simulink model "aerosonde_dynamics_with_autopilot"  (R2021b)
settings: Solver=ode3  StartTime=0.0  StopTime=250  FixedStep=dt  RelTol=1e-6  EnableMultiTasking=on
InitFcn:
  | aerosonde_initialize
  | fault_configurations
  | init_sensor_model
StopFcn:
  | aerosende_grafik;
values from neighbouring files (symbols this model uses):
  aerosonde = AircraftSimData    [aerosonde_data.m]    (also in aerosonde_initialize.m = aerosonde_data)
  aoa_sensor_measurement_limit_rad = deg2rad(30)    [init_sensor_model.m]
  aoa_sensor_noise_power = 0.00030462    [init_sensor_model.m]
  bias_fault_active = TRUE    (= 1)    [fault_configurations.m]
  bias_fault_time = 150    [fault_configurations.m]
  bias_rad = deg2rad(3)    [fault_configurations.m]
  drift_fault_active = FALSE    (= 0)    [fault_configurations.m]
  drift_limit_rad = deg2rad(20)    [fault_configurations.m]
  drift_ratio_rad_s = deg2rad(0.2)    [fault_configurations.m]
  dt = 1/50    (= 0.02)    [aerosonde_initialize.m]
  F = [0 1 0 ... (first row only)    [aerosonde_initialize.m]
  flightconfig = flightconfig_data    [aerosonde_initialize.m]    (also in flightconfig_data.m = siminitialdetails)
  stuck_fault_active = FALSE    (= 0)    [fault_configurations.m]
  x_init = [510.0; -flightconfig.We_VL  ; 0.0]    [aerosonde_initialize.m]
undefined symbols (not defined in the file or in its folder): magnitude, MIL
libraries: simulink_extras x24, simulink x6, aerolibasang x3, aerolibwind2 x3, aerolibbdyn x2, aerolibadyn x1, aerolibtransform2 x1, shareddyn x1, aerolibobsolete x1, sharedutil x1, aerolibatmos2 x1
(part 1 of 2)
settings Model: PacingRate=10  ExtModeTrigDuration=100  Creator=eh3081  LastModifiedBy=altin
settings SolverCC: AlgebraicLoopSolver=TrustRegion
settings DataIOCC: SaveFormat=Array  SignalLoggingSaveFormat=ModelDataLogs  SaveOutput=off  SignalLogging=off  DSMLogging=off  SaveTime=off  StateSaveName=tmp_raccel_xout  SignalLoggingName=tmp_raccel_logsout
settings OptimizationCC: ExpressionDepthLimit=2147483647  InitFltsAndDblsToZero=on  EfficientMapNaN2IntZero=off  LifeSpan=inf
settings DebuggingCC: ReadBeforeWriteMsg=DisableAll  WriteAfterWriteMsg=DisableAll  WriteAfterReadMsg=DisableAll  AlgebraicLoopMsg=none  SaveWithParameterizedLinksMsg=none  UnderspecifiedInitializationDetection=Classic  MergeDetectMultiDrivingBlocksExec=none  SolverPrmCheckMsg=warning  MultiTaskDSMMsg=warning  MultiTaskCondExecSysMsg=none  StateNameClashWarn=warning  SFUnexpectedBacktrackingDiag=warning  SFNoUnconditionalDefaultTransitionDiag=warning  SFExecutionAtInitializationDiag=none  SFMachineParentedDataDiag=warning  ArithmeticOperatorsInVariantConditions=warning
settings HardwareCC: ProdBitPerPointer=32  ProdBitPerSizeT=32  ProdBitPerPtrDiffT=32  ProdLargestAtomicFloat=None  ProdIntDivRoundTo=Undefined  ProdEndianess=Unspecified  ProdWordSize=32  ProdHWDeviceType=32-bit Generic  TargetBitPerPointer=64  TargetBitPerSizeT=64  TargetBitPerPtrDiffT=64  TargetLongLongMode=on  TargetIntDivRoundTo=Zero  TargetEndianess=LittleEndian  TargetWordSize=64  TargetHWDeviceType=MATLAB Host  ProdEqTarget=off
settings ModelReferenceCC: UpdateModelReferenceTargets=IfOutOfDate  PropagateSignalLabelsOutOfModel=off
settings SFSimCC: SFSimEcho=off  SimUseLocalCustomCode=off  CustomCodeUndefinedFunction=UseInterfaceOnly
settings RTWCC: SystemTargetFile=raccel.tlc  TemplateMakefile=raccel_default_tmf  RTWVerbose=off  RTWUseLocalCustomCode=off  RTWUseSimCustomCode=on
settings CodeAppCC: GenerateComments=off  MaxIdLength=128  MangleLength=10  SimulinkBlockComments=off
settings RaccelTargetCC: ParMdlRefBuildCompliant=off  ENABLE_SLEXEC_SSBRIDGE=0  RTWCAPISignals=off  RTWCAPIParams=off  RTWCAPIRootIO=off
settings ConfigComp: CovMetricSettings=dw  CovSaveCumulativeToWorkspaceVar=on  CovSaveSingleToWorkspaceVar=on  CovExternalEMLEnable=off
settings SimscapeCC: SimscapeNormalizeSystem=off
settings ConfigurationSet: Description=SimMechanics 2G

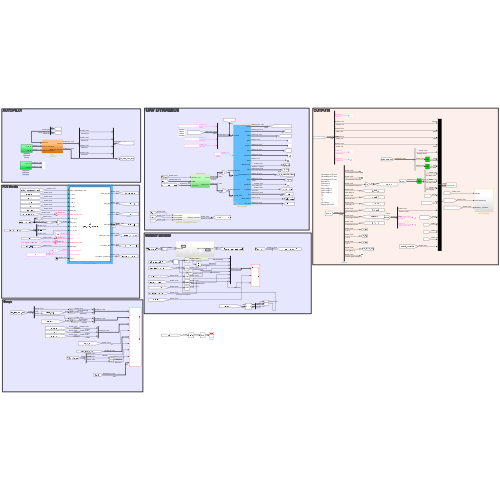
[thumbnail: Simulink's stored preview of the top-level diagram]
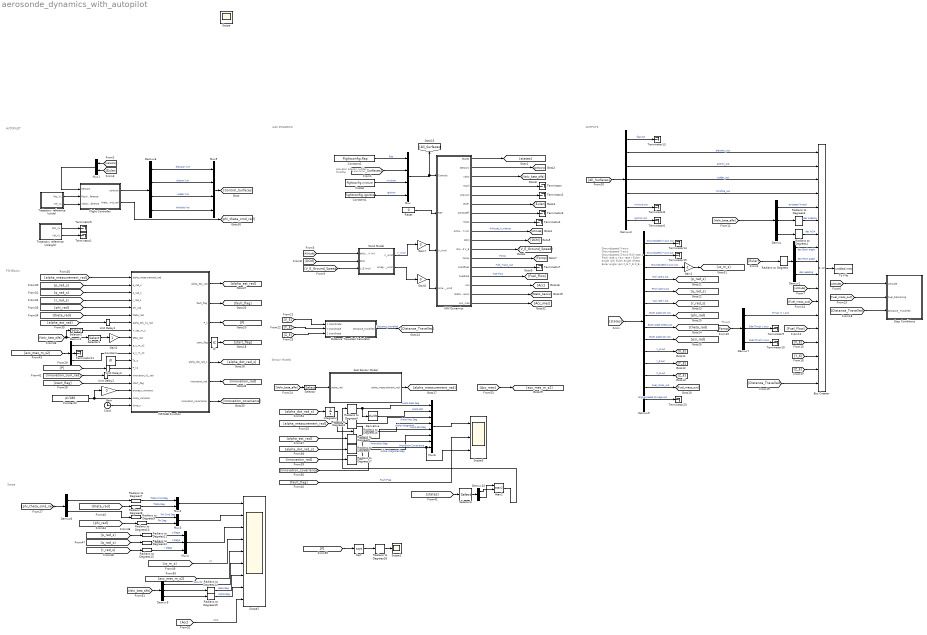
== system aerosonde_dynamics_with_autopilot ==
  note: Scope
  note: FDI Blocks
  note: Sensor Models
  note: AUTOPILOT
  note: OUTPUTS
  note: UAV DYNAMICS
  note: Thrust
  note: elevator
      | aileron
      | rudder
      | throttle
  note: Groundspeed X-axis
      | Groundspeed Y-axis
      | Groundspeed Z-axis
      | Roll rate p
      | Pitch rate q
      | Yaw rate r
      | Euler angle \phi
      | Euler angle \theta
      | Euler angle \psi
      | X_E
      | Y_E
      | Z_E
      | Fuel mass
      | Engine speed \Omega
  " UAV Dynamics" : Subsystem  mask(6-DOF Aerosonde Model){as=aerosonde, Velocities0=flightconfig.velocity_0, Rates0=flightconfig.rates_0, Euler0=flightconfig.euler_0, Position0=flightconfig.position_0, Fuel0=flightconfig.fuel_0, Omega0=flightconfig.Omega_0, GndAlt=0}
      mask prompts: as "Aircraft configuration data:"; Velocities0 "Initial velocity in body axes [u,v,w]: (m/s)"; Rates0 "Initial body rotation rates [p,q,r]: (rad/s)"; Euler0 "Initial Euler orientation [roll, pitch, yaw]: (rad)"; Position0 "Initial position in inertial axes [Xe,Ye,Ze]: (m)"; Fuel0 "Initial fuel mass: (Kg)"; Omega0 "Initial engine speed: (rad/s)"; GndAlt "Ground altitude: (m)"
      mask help:
      | Nonlinear 6-DOF Aerosonde  model with equations of motion in
      | body frame.
      |
      | Version 2011a (18 February 2011)
      mask Help:
      | The block implements the 6-DOF nonlinear Aerosonde model. It is an adaptation of the model provided in the AeroSim blockset. Velocities are computed in body frame.
      | <P><B>Inputs:</B>
      | <LI>Controls = the 4x1 vector of aircraft controls [elevator aileron rudder throttle]. Aerodynamic controls are in radians, throttle is from 0 to 1.</LI>
      | <LI>RST = the integrator reset flag (0 or 1, all integrators on rising edge)
      | <LI>V_wind = the 3x1 vector of background wind speed components in navigation frame [North East Down]</LI>
      | <LI>omega_wind = the 3x1 vector of background wind angular rates in navigation frame [North East Down]</LI>
      | </P>
      | <P><B>Outputs:</B>
      | <LI>States = the 14x1 aircraft state vector [Velocities, Angular rates, Euler angles, Position, Fuel mass, Engine speed].</LI>
      | <LI>Sensors = the 15x1 vector of sensor outputs [GPS Position, GPS Groundspeed, Accelerometers, Gyros, Air data].</LI>
      | <LI>VelW = the 3x1 vector of aircraft velocity in wind axes [Airspeed, sideslip, angle of attack]</LI>
      | <LI>Mach = the Mach number</LI>
      | <LI>Ang Acc = the 3x1 vector of angular accelerations
      | <LI>Euler = the 3x1 vector of Euler angles (roll, pitch, yaw)</LI>
      | <LI>AeroCoeff = the 6x1 vector of aerodynamic coefficients [CD CY CL Cl Cm Cn]</LI>
      | <LI>Mass = the current aircraft mass</LI>
      | <LI>h = the aircraft altitude</LI>
      | </P>
      | <P><B>Parameters:</B>
      | <LI>Aircraft configuration data = structured varaible with aircraft data<BR>
      | obtain by  ``aerosonde=aerosonde_initialize'' for example</LI>
      | <LI>Initial velocities = the 3x1 vector of initial aircraft velocities in body axes [u v w]</LI>
      | <LI>Initial angular rates = the 3x1 vector of initial angular rates [p q r]</LI>
      | <LI>Initial attitude = the 3x1 vector of initial Euler angles [phi theta psi]</LI>
      | <LI>Initial position = the 3x1 vector of initial aircraft location [Lat Lon Alt]</LI>
      | <LI>Initial fuel mass = the initial quantity of fuel on-board the aircraft</LI>
      | <LI>Initial engine speed = the initial engine rotation speed</LI>
      | <LI>Ground altitude = the ground altitude at aircraft location</LI>
      | </P>
      | <P>
      | <I>Version 2010b (26 May 2010)</I>
      | </P>
  AoA Sensor Model : Subsystem
  Atan2 : Trigonometry  Operator=atan2
  Bus Creator : BusCreator  Inputs=18
  Clock : Clock
  Constant : Constant  Value=dt
  Constant1 : Constant  Value=flightconfig.ignition
  Constant2 : Constant  Value=flightconfig.flap
  Constant3 : Constant  Value=pi/180
  Costat : Constant  Value=flightconfig.mixture
  Demux{,1..2,7,9} (5 alike) : Demux  Outputs=3
      Demux settings: DisplayOption=none
      Demux1 settings: DisplayOption=none
  Demux10 : Demux  Outputs=2
  Demux3 : Demux  Outputs=7
  Demux5 : Demux  Outputs=14
  Demux6 : Demux
  Demux8 : Demux  Outputs=2
  Derivative : Derivative
  Distance Travelled Calculator : Subsystem
  Flight Controller : Subsystem
  Gain : Gain  Gain=0
  Gain1 : Gain  Gain=-1
  Gain2 : Gain
  Gain6 : Gain  Gain=0
  Gain7 : Gain  Gain=0
  IC : InitialCondition
  Integrator : Integrator
  MATLAB Function : MATLAB Function  TreatAsAtomicUnit=on
  Mux : Mux  Inputs=[1 4 1 1]
  Mux1 : Mux  Inputs=[15 3]
  Mux2 : Mux  Inputs=2
  Mux3 : Mux  Inputs=2
  Mux4 : Mux  Inputs=3
  Mux5 : Mux
  Mux6 : Mux  Inputs=8
  Radians to Degrees{,1..18} (19 alike) : simulink_extras/Transformations/Radians to Degrees
  Reset : Constant  Value=0
  Scope1 : Scope
  Scope2 : Scope  NumInputPorts=9
  Scope3 : Scope  NumInputPorts=3
  Selector : Selector  InputPortWidth=3  IndexOptions=Index vector (dialog)  Indices=[3]  OutputSizes=1
  Selector1 : Selector  InputPortWidth=3  IndexOptions=Index vector (dialog)  Indices=[2]  OutputSizes=1
  Selector2 : Selector  InputPortWidth=3  IndexOptions=Index vector (dialog)  Indices=[1]  OutputSizes=1
  Selector3 : Selector  InputPortWidth=14  IndexOptions=Index vector (dialog)  Indices=[1 3]  OutputSizes=1
  Sqrt : Sqrt  SaturateOnIntegerOverflow=on
  Stop Conditions : Subsystem
  Terminator{,1..11,13..15,23} (16 alike) : Terminator
  To File : ToFile  MatrixName=fdm  SaveFormat=Timeseries
      settings: Decimation=flightconfig.decimationlogging
  Trajectory reference (circle) : Subsystem
  Trajectory reference (straight) : Subsystem
  Unit Delay1 : UnitDelay  SampleTime=-1  HasFrameUpgradeWarning=on
  Unit Delay2 : UnitDelay  SampleTime=-1  HasFrameUpgradeWarning=on
  Unit Delay3 : UnitDelay  InitialCondition=1e-3  SampleTime=-1  HasFrameUpgradeWarning=on
  Wind Model : Subsystem
  Scope : Scope
  wires:
  Reset/1 -> " UAV Dynamics"/2(RST)
  " UAV Dynamics"/1(States) -> [states]
  Demux/3 -> Radians to Degrees1/1
  Demux/2 -> Radians to Degrees2/1
  Demux/1 -> Bus Creator/5  "airspeed (knots)"
  Radians to Degrees2/1 -> Bus Creator/6  "dec sideslip"
  Radians to Degrees1/1 -> Bus Creator/7  "dec AOA"
  Radians to Degrees/1 -> Demux1/1
  Demux1/2 -> Bus Creator/9  "dec Pitch angle"
  Demux1/3 -> Bus Creator/10  "dec Heading"
  Demux1/1 -> Bus Creator/8  "dec Bank angle"
  Wind Model/1(V_wind) -> Gain7/1  "V_wind"
  Wind Model/2(omega_wind) -> Gain6/1
  " UAV Dynamics"/4(Mach) -> Terminator/1
  " UAV Dynamics"/5(Ang Acc) -> Terminator2/1
  " UAV Dynamics"/7(AeroCoeff) -> Terminator3/1
  " UAV Dynamics"/8(Mass) -> Terminator4/1
  Constant2/1 -> Mux/1  "flap"
  Costat/1 -> Mux/3  "mixture"
  Constant1/1 -> Mux/4  "ignition"
  Mux/1 -> [All_Surfaces], " UAV Dynamics"/1(Controls)
  Flight Controller/1(controls) -> Demux6/1
  Mux1/1 -> Flight Controller/1(Sensors)
  [states] -> Demux5/1
  Trajectory reference (straight)/2(Vel_VL) -> Terminator1/1
  Trajectory reference (straight)/1(Pos_VL) -> Terminator5/1
  Trajectory reference (circle)/2(Vel_VL) -> Flight Controller/3(Velocity reference)
  Demux3/1 -> Terminator13/1  "flap out"
  Demux3/6 -> Terminator8/1  "mixture out"
  Demux3/7 -> Terminator6/1  "ignition out"
  Demux5/1 -> Terminator14/1  "Groundspeed X-axis out"
  Demux5/14 -> Terminator23/1  "Engine speed \\Omega out"
  Demux5/9 -> [psi_rad]  "Euler angle \\psi out"
  Demux5/8 -> [theta_rad]  "Euler angle \\theta out"
  Demux5/7 -> [phi_rad]  "Euler angle \\phi out"
  Demux5/6 -> [r_rad_s]  "Yaw rate r out"
  Demux5/2 -> Terminator15/1  "Groundspeed Y-axis out"
  Demux5/3 -> Gain1/1  "Groundspeed Z-axis out"
  Demux5/4 -> [p_rad_s]  "Roll rate p out"
  Demux5/5 -> [q_rad_s]  "Pitch rate q out"
  Demux5/10 -> [X_E]  "X_E out"
  Demux5/12 -> [Z_E]  "Z_E out"
  Demux6/1 -> Mux5/1  "elevator live"
  Demux6/3 -> Mux5/3  "rudder live"
  Demux6/4 -> Mux5/4  "throttle live"
  Demux7/1 -> Bus Creator/13  "Thrust in x axis"
  Demux7/2 -> Terminator9/1  "Side Thrust y axis"
  Demux7/3 -> Terminator10/1  "Side Thrust z axis"
  Bus Creator/1 -> To File/1
  " UAV Dynamics"/9("Altitude h (m) ") -> [Altitude]  "Altitude_h_metres"
  " UAV Dynamics"/13(OutofFuel) -> Terminator7/1  "Fuel_mass_out"
  Demux3/2 -> Bus Creator/1  "elevator_out"
  Demux3/3 -> Bus Creator/2  "aileron_out"
  Demux3/4 -> Bus Creator/3  "rudder_out"
  Demux3/5 -> Bus Creator/4  "throttle_out"
  Demux5/11 -> [Y_E]  "Y_E out"
  Demux6/2 -> Mux5/2  "aileron live"
  Mux5/1 -> [Control_Surfaces]
  [Control_Surfaces] -> Mux/2
  " UAV Dynamics"/2(Sensors) -> [sensors]
  [sensors] -> Mux1/1
  [Euler] -> Mux1/2
  " UAV Dynamics"/6(Euler) -> [Euler]
  [Euler] -> Radians to Degrees/1
  [Altitude] -> Wind Model/1(altitude h (m))
  [Altitude] -> Bus Creator/11
  [Altitude] -> Stop Conditions/1(Altitude)
  " UAV Dynamics"/10(DCM) -> [DCM]
  [DCM] -> Wind Model/2(DCM)
  " UAV Dynamics"/11(Groundspeed V_E) -> [V_E_Ground_Speed]
  [V_E_Ground_Speed] -> Wind Model/3(V_E (m/s))
  " UAV Dynamics"/12(Fprop) -> [Fprop]  "Fprop"
  [Fprop] -> Demux7/1
  " UAV Dynamics"/3(VelW) -> [Velw_beta_alfa]
  [Velw_beta_alfa] -> Demux/1
  " UAV Dynamics"/14(FuelRate) -> [Fuel_Flow]  "Fuel Flow"
  [Fuel_Flow] -> Bus Creator/14
  Demux5/13 -> [Fuel_mass_out]  "Fuel_mass_out"
  [Fuel_mass_out] -> Stop Conditions/2(Fuel_Remaining)
  [Fuel_mass_out] -> Bus Creator/12
  [X_E] -> Bus Creator/15
  [Y_E] -> Bus Creator/16
  [Z_E] -> Bus Creator/17
  Distance Travelled Calculator/1(Distance_travelled) -> [Distance_Travelled]  "Distance_travelled"
  [Distance_Travelled] -> Stop Conditions/3(Distance_ Travelled)
  [Distance_Travelled] -> Bus Creator/18
  [All_Surfaces] -> Demux3/1
  [X_E] -> Distance Travelled Calculator/1(X Coordinate)
  [Y_E] -> Distance Travelled Calculator/2(Y Coordinate)
  [Z_E] -> Distance Travelled Calculator/3(Z coordinate)
  Trajectory reference (circle)/1(Pos_VL) -> Flight Controller/2(Position reference)
  " UAV Dynamics"/15(" Acc") -> [Acc]
  " UAV Dynamics"/16(Statik_Basinc) -> [Statik_basinc]
  Gain6/1 -> " UAV Dynamics"/4(omega_wind)
  Gain7/1 -> " UAV Dynamics"/3(V_wind)
  [Velw_beta_alfa] -> Selector/1
  Selector/1 -> AoA Sensor Model/1(alpha_rad)
  AoA Sensor Model/1(alpha_measurement_rad) -> [alpha_measurement_rad]
  [alpha_measurement_rad] -> Radians to Degrees3/1
  Radians to Degrees3/1 -> Mux6/3  "Alpha Mes Deg"
  Radians to Degrees4/1 -> Mux6/1, Derivative/1  "Alpha Real Deg"
  [alpha_measurement_rad] -> MATLAB Function/1(alpha_measurement_rad)
  [acc_mes_m_s2] -> Demux2/1
  Demux2/1 -> MATLAB Function/10(a_x_m_s2)
  Demux2/3 -> MATLAB Function/11(a_z_m_s2)
  Constant/1 -> MATLAB Function/12(Ts_s)
  MATLAB Function/4(start_flag) -> IC/1
  IC/1 -> [start_flag]
  [start_flag] -> MATLAB Function/15("start_flag ")
  [P] -> Unit Delay3/1
  Gain/1 -> MATLAB Function/16(process_variance)
  Constant3/1 -> Gain/1, MATLAB Function/17(noise_variance)
  [p_rad_s] -> MATLAB Function/2(p_rad_s)
  [q_rad_s] -> MATLAB Function/3(q_rad_s)
  [r_rad_s] -> MATLAB Function/4(r_rad_s)
  [phi_rad] -> MATLAB Function/5(phi_rad)
  [alpha_est_rad] -> Unit Delay1/1
  MATLAB Function/1(alpha_est_rad) -> [alpha_est_rad]
  MATLAB Function/2(fault_flag) -> [fault_flag]
  [alpha_est_rad] -> Radians to Degrees5/1
  Radians to Degrees5/1 -> Mux6/5  "Alpha Est Deg"
  MATLAB Function/5(alpha_dot_rad_s) -> [alpha_dot_rad_s]
  [alpha_dot_rad_s] -> Radians to Degrees6/1
  Radians to Degrees6/1 -> Mux6/6  "Alpha Integrated Deg"
  Unit Delay1/1 -> MATLAB Function/7(alpha_est_k1_rad)
  [Velw_beta_alfa] -> Selector1/1, Selector2/1
  Selector2/1 -> MATLAB Function/8(V_tas_m_s)
  Demux2/2 -> Terminator11/1
  Selector1/1 -> Gain2/1
  Flight Controller/2(theta_phi_cmd_rad) -> [phi_theta_cmd_rad]
  [phi_theta_cmd_rad] -> Demux8/1
  Demux8/1 -> Radians to Degrees7/1
  Radians to Degrees7/1 -> Mux2/1  "Theta Cmd Deg"
  Radians to Degrees8/1 -> Mux2/2  "Theta Deg"
  Mux2/1 -> Scope2/1
  [theta_rad] -> Radians to Degrees8/1
  Demux8/2 -> Radians to Degrees9/1
  [phi_rad] -> Radians to Degrees10/1
  Radians to Degrees9/1 -> Mux3/1  "Phi Cmd Deg"
  Mux3/1 -> Scope2/2
  [p_rad_s] -> Radians to Degrees11/1
  Radians to Degrees10/1 -> Mux3/2  "Phi Deg"
  [r_rad_s] -> Radians to Degrees13/1
  [q_rad_s] -> Radians to Degrees12/1
  Radians to Degrees11/1 -> Mux4/1  "p Deg/s"
  Radians to Degrees12/1 -> Mux4/2  "q Deg/s"
  Radians to Degrees13/1 -> Mux4/3  "r Deg/s"
  Mux4/1 -> Scope2/3
  Gain1/1 -> [vz_m_s]
  [vz_m_s] -> Scope2/4  "Vz"
  Gain2/1 -> MATLAB Function/9(beta_rad)
  Clock/1 -> MATLAB Function/18(time_s)
  [acc_mes_m_s2] -> Scope2/5
  [Velw_beta_alfa] -> Demux9/1
  Demux9/1 -> Scope2/6  "TAS Kts"
  Demux9/2 -> Radians to Degrees14/1
  Demux9/3 -> Radians to Degrees15/1
  Radians to Degrees14/1 -> Scope2/7  "Beta Deg"
  Radians to Degrees15/1 -> Scope2/8  "Alpha Deg"
  [Acc] -> Scope2/9  "ACC"
  [states] -> Selector3/1
  Selector3/1 -> Demux10/1
  Demux10/2 -> Atan2/1
  Demux10/1 -> Atan2/2
  Atan2/1 -> Radians to Degrees4/1
  " UAV Dynamics"/17(Acc_mes) -> [Acc_mes]
  [Acc_mes] -> [acc_mes_m_s2]
  Derivative/1 -> Mux6/2  "Alpha Dot"
  [alpha_dot_rad_s] -> Integrator/1
  Integrator/1 -> Radians to Degrees16/1
  Radians to Degrees16/1 -> Mux6/4  "Alpha Integrated"
  MATLAB Function/6(innovation_rad) -> [innovation_rad]
  [innovation_rad] -> Radians to Degrees17/1
  Radians to Degrees17/1 -> Mux6/7  "Innovaiton Deg"
  Mux6/1 -> Scope3/1
  [fault_flag] -> Scope3/2  "Fault Flag"
  [innovation_cum_rad] -> Unit Delay2/1
  Unit Delay2/1 -> MATLAB Function/14(innovation_k1_rad)
  MATLAB Function/7(innovation_covariance) -> [innovation_covariance]
  [innovation_covariance] -> Scope3/3, Mux6/8  "Innovaiton Covariance"
  MATLAB Function/3(P_k) -> [P]
  [P] -> Sqrt/1
  [theta_rad] -> MATLAB Function/6(theta_rad)
  Unit Delay3/1 -> MATLAB Function/13(P_k1)
  Radians to Degrees18/1 -> Scope1/1
  Sqrt/1 -> Radians to Degrees18/1

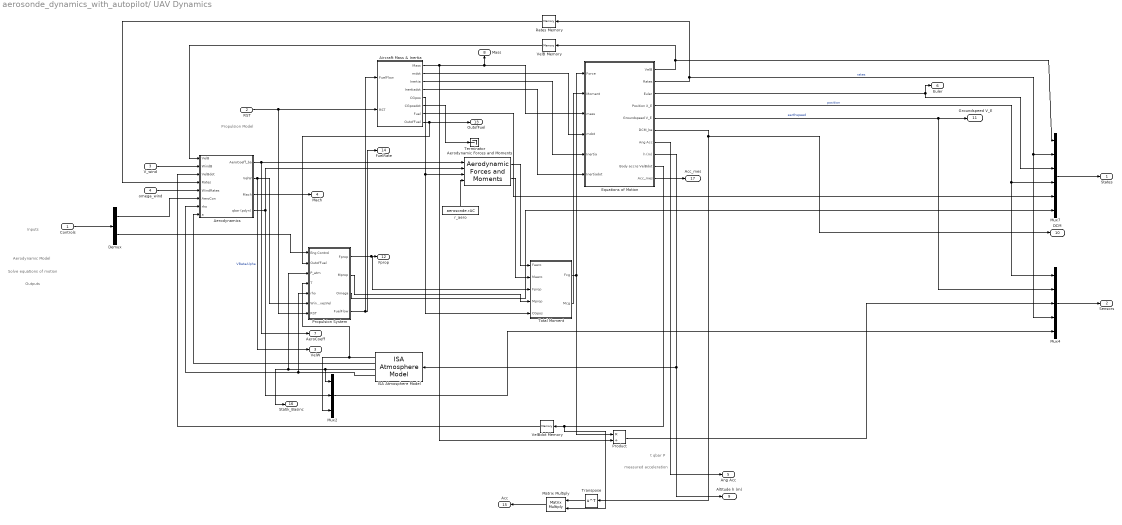
== system aerosonde_dynamics_with_autopilot/ UAV Dynamics ==
  note: t qbar P
  note: measured acceleration
  note: Propulsion Model
  note: Aerodynamic Model
  note: Outputs
  note: Inputs
  note: Solve equations of motion
  Controls : Inport
  RST : Inport  Port=2
  V_wind : Inport  Port=3
  omega_wind : Inport  Port=4
  Aerodynamic Forces and Moments : aerolibadyn/Aerodynamic Forces and Moments   inputAxes=Body  outputForceAxes=Body  outputMomentAxes=Body  S=aerosonde.S  b=aerosonde.b  cbar=aerosonde.c
  Aerodynamics : Subsystem
  Aircraft Mass & Inertia : Subsystem
  Demux : Demux  Outputs=[4,3]
      settings: DisplayOption=none
  Equations of Motion : Subsystem
  ISA Atmosphere Model : aerolibatmos2/ISA Atmosphere Model  custom=off  g=9.80665  gamma=1.4  R=287.0531  L=0.0065  h_trop=11000  h_strat=20000  rho0=1.225  P0=101325  T0=288.15  h0=0
  Matrix Multiply : Product  Multiplication=Matrix(*)
  Mux2 : Mux  Inputs=3
  Mux4 : Mux  Inputs=5
  Mux7 : Mux  Inputs=6
  Product : Product  Inputs=*/  RndMeth=Zero
  Propulsion System : Subsystem  mask(General-aviation propulsion system){OmegaIni=Omega0, RPM=aerosonde.RPM, MAP=aerosonde.MAP, FuelFlow=aerosonde.pFuelFlow, Power=aerosonde.Power, Jeng=aerosonde.Jeng, J=aerosonde.J, CT=aerosonde.CT, CP=aerosonde.CP, Rprop=aerosonde.Rprop, Jprop=aerosonde.Jprop, TSL=aerosonde.TSL}
      mask prompts: OmegaIni "Initial engine speed:"; RPM "Engine RPM vector:"; MAP "Engine MAP vector:"; FuelFlow "Engine fuel flow look-up table:"; Power "Engine power look-up table:"; Jeng "Engine moment of inertia:"; J "Propeller advance ratio vector:"; CT "Propeller coefficient of thrust vector:"; CP "Propeller coefficient of power vector:"; Rprop "Propeller radius:"; Jprop "Propeller moment of inertia:"; TSL "Sea-level temperature:"
      mask help: The block models a general aviation propulsion system including a piston engine and a fixed-pitch propeller.
      mask Help:
      | The block provides a general aviation propulsion system using the AeroSim piston engine and fixed-pitch propeller models.
      | <P><B>Inputs:</B>
      | <LI>Control = the 3x1 engine control vector [Throttle Mixture Ignition]</LI>
      | <LI>OutofFuel = the out-of-fuel flag (0 or 1)</LI>
      | <LI>p = the static pressure at current altitude, in Pa</LI>
      | <LI>T = the air temperature at current altitude, in K</LI>
      | <LI>rho = the air density at current altitude, in kg/m^3</LI>
      | <LI>WindAxesVel = the 3x1 vector of body velocities in wind axes [Airspeed Sideslip Angle-of-attack] in [m/s rad rad]</LI>
      | <LI>RST = the integrator reset flag (rising edge)</LI>
      | </P>
      | <P><B>Output:</B>
      | <LI>Fprop = the 3x1 vector of propulsion system forces applied to the airframe, at the propeller hub location</LI>
      | <LI>Mprop = the 3x1 vector of propulsion system moments applied to the airframe</LI>
      | <LI>Omega = the engine shaft rotation speed, in rad/s</LI>
      | <LI>FuelFlow = the mass fuel flow, in kg/s</LI>
      | <LI>EngCoeff = the 5x1 engine coefficient vector [MAP Airflow Fuelflow BSFC Power] in [kPa kg/s kg/s g/(W*hr) W]</LI>
      | <LI>PropCoeff = the 3x1 propeller coefficient vector [J CT CP]</LI>
      | </P>
      | <P><B>Parameters:</B>
      | <LI>Initial engine speed = the initial value for the engine speed, in rad/s</LI>
      | <LI>RPM vector = the engine speed interpolation vector, in rpm</LI>
      | <LI>MAP vector = the manifold air pressure interpolation vector, in kPa</LI>
      | <LI>Fuel flow = the 2-D look-up table for fuel flow, as function of MAP and RPM, in g/hr</LI>
      | <LI>Power = the 2-D look-up table for power, as function of MAP and RPM, in W</LI>
      | <LI>Engine moment of inertia = the moment of inertia of the rotating engine parts (shaft)</LI>
      | <LI>Advance ratio = the advance ratio vector for interpolation</LI>
      | <LI>Coefficient of thrust = the coefficient of thrust vector for interpolation</LI>
      | <LI>Coefficient of power = the coefficient of power vector for interpolation</LI>
      | <LI>Radius = the propeller radius</LI>
      | <LI>Propeller moment of inertia = the moment of inertia of the propeller</LI>
      | <LI>Sea-level temperature = the ambient temperature for which the above engine look-up tables are given</LI>
      | </P>
  Rates Memory : Memory  InitialCondition=flightconfig.rates_0  LinearizeMemory=on
  Terminator : Terminator
  Total Moment : Subsystem
  Transpose : Math  Operator=transpose  SaturateOnIntegerOverflow=on
  VelB Memory : Memory  InitialCondition=flightconfig.velocity_0  LinearizeMemory=on
  VelBdot Memory : Memory  LinearizeMemory=on
  r_aero : Constant  Value=aerosonde.rAC
  States : Outport
  Sensors : Outport  Port=2
  VelW : Outport  Port=3
  Mach : Outport  Port=4
  Ang Acc : Outport  Port=5
  Euler : Outport  Port=6
  AeroCoeff : Outport  Port=7
  Mass : Outport  Port=8
  "Altitude h (m) " : Outport  Port=9
  DCM : Outport  Port=10
  Groundspeed V_E : Outport  Port=11
  Fprop : Outport  Port=12
  OutofFuel : Outport  Port=13  OutDataTypeStr=boolean
  FuelRate : Outport  Port=14
  " Acc" : Outport  Port=15
  Statik_Basinc : Outport  Port=16
  Acc_mes : Outport  Port=17
  wires:
  Aircraft Mass & Inertia/7(Fuel) -> Mux7/5
  Propulsion System/3(Omega) -> Mux7/6
  ISA Atmosphere Model/4 -> Propulsion System/5(rho), Aerodynamics/7(rho)
  VelB Memory/1 -> Aerodynamics/1(VelB)
  Equations of Motion/6(DCM_be) -> Transpose/1, DCM/1
  Rates Memory/1 -> Aerodynamics/4(Rates)
  Equations of Motion/1(VelB) -> VelB Memory/1, Mux7/1
  Mux4/1 -> Sensors/1
  VelBdot Memory/1 -> Aerodynamics/3(VelBdot)
  Aerodynamic Forces and Moments/1 -> Total Moment/1(Faero)
  Equations of Motion/7(Ang Acc) -> Ang Acc/1
  Mux2/1 -> Mux4/5
  Aerodynamics/2(VelW) -> VelW/1, Propulsion System/6(WindAxesVel)  "VBetaAlpha"
  omega_wind/1 -> Aerodynamics/5(WindRates)
  Propulsion System/2(Mprop) -> Total Moment/4(Mprop)
  Equations of Motion/5(Groundspeed V_E) -> Mux4/2, Groundspeed V_E/1  "earthspeed"
  Total Moment/2(Mcg) -> Equations of Motion/2(Moment)
  Equations of Motion/4(Position X_E) -> Mux4/1, Mux7/4  "position"
  Controls/1 -> Demux/1
  Mux7/1 -> States/1
  Demux/2 -> Propulsion System/1(Eng Control)
  Demux/1 -> Aerodynamics/6(AeroCon)
  Aerodynamic Forces and Moments/2 -> Total Moment/2(Maero)
  Aerodynamics/3(Mach) -> Mach/1
  ISA Atmosphere Model/2 -> Aerodynamics/8("a ")
  Aircraft Mass & Inertia/2(mdot) -> Equations of Motion/4(mdot)
  r_aero/1 -> Aerodynamic Forces and Moments/4
  Aircraft Mass & Inertia/3(Inertia) -> Equations of Motion/5(Inertia)
  Aircraft Mass & Inertia/4(Inertiadot) -> Equations of Motion/6(Inertiadot)
  RST/1 -> Aircraft Mass & Inertia/2(RST), Propulsion System/7(RST)
  Aircraft Mass & Inertia/6(CGposdot) -> Terminator/1
  Product/1 -> Mux4/3
  Equations of Motion/9(Body accns VelBdot) -> Matrix Multiply/2, VelBdot Memory/1
  Aerodynamics/1(AeroCoeff_ba) -> Aerodynamic Forces and Moments/1, AeroCoeff/1
  V_wind/1 -> Aerodynamics/2(WindB)
  Equations of Motion/3(Euler) -> Mux7/3, Euler/1
  Aircraft Mass & Inertia/8(OutofFuel) -> OutofFuel/1, Propulsion System/2(OutofFuel)
  Aircraft Mass & Inertia/5(CGpos) -> Aerodynamic Forces and Moments/3, Total Moment/5(CGpos)
  Aerodynamics/4(qbar (pdyn)) -> Aerodynamic Forces and Moments/2, Mux2/2
  Propulsion System/1(Fprop) -> Fprop/1, Total Moment/3(Fprop)
  Aircraft Mass & Inertia/1(Mass) -> Equations of Motion/3(mass), Mass/1, Product/2
  Equations of Motion/2(Rates) -> Mux4/4, Mux7/2, Rates Memory/1  "rates"
  ISA Atmosphere Model/1 -> Mux2/3, Propulsion System/4(T)
  ISA Atmosphere Model/3 -> Mux2/1, Statik_Basinc/1, Propulsion System/3(P_atm)
  Equations of Motion/8(h (m)) -> "Altitude h (m) "/1, ISA Atmosphere Model/1
  Total Moment/1(Fcg) -> Product/1, Equations of Motion/1(Force)
  Propulsion System/4(FuelFlow) -> FuelRate/1, Aircraft Mass & Inertia/1(FuelFlow)
  Transpose/1 -> Matrix Multiply/1
  Matrix Multiply/1 -> " Acc"/1
  Equations of Motion/10(Acc_mes) -> Acc_mes/1

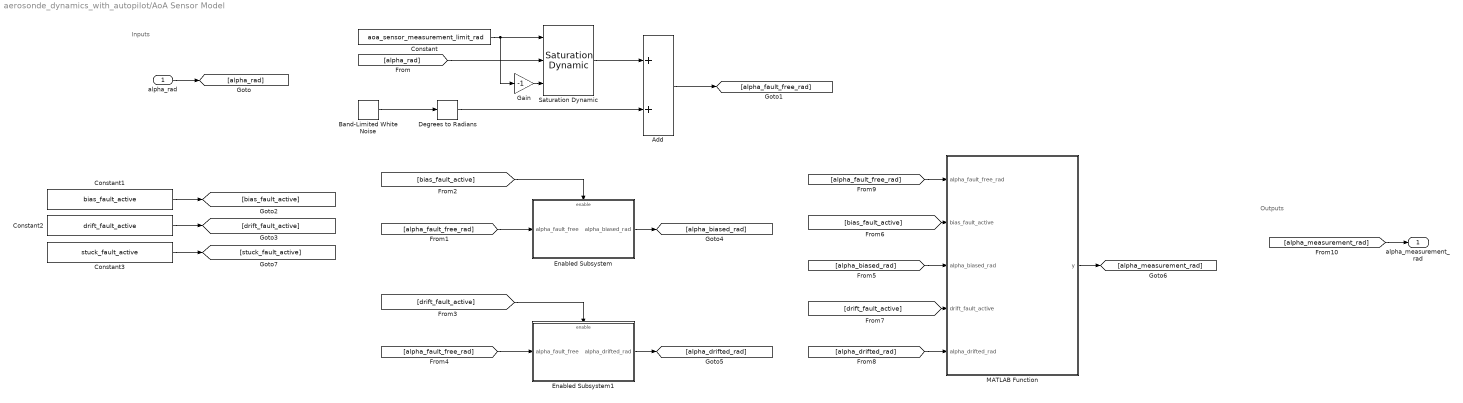
== system aerosonde_dynamics_with_autopilot/AoA Sensor Model ==
  note: Outputs
  note: Inputs
  alpha_rad : Inport
  Add : Sum
  Band-Limited White Noise : simulink/Sources/Band-Limited White Noise  Cov=[aoa_sensor_noise_power]  Ts=dt  seed=[23341]
  Constant : Constant  Value=aoa_sensor_measurement_limit_rad
  Constant1 : Constant  Value=bias_fault_active
  Constant2 : Constant  Value=drift_fault_active
  Constant3 : Constant  Value=stuck_fault_active
  Degrees to Radians : simulink_extras/Transformations/Degrees to Radians
  Enabled Subsystem : Subsystem  TreatAsAtomicUnit=on
  Enabled Subsystem1 : Subsystem  TreatAsAtomicUnit=on
  Gain : Gain  Gain=-1
  MATLAB Function : MATLAB Function  TreatAsAtomicUnit=on
  Saturation Dynamic : simulink/Discontinuities/Saturation Dynamic  OutMin=[]  OutMax=[]  OutDataTypeStr=Inherit: Same as second input  OutDataType=fixdt(1, 16)  OutScaling=2^-10  DoSatur=off
  alpha_measurement_rad : Outport
  wires:
  alpha_rad/1 -> [alpha_rad]
  [alpha_rad] -> Saturation Dynamic/2
  Gain/1 -> Saturation Dynamic/3
  Constant/1 -> Saturation Dynamic/1, Gain/1
  Saturation Dynamic/1 -> Add/1
  Band-Limited White Noise/1 -> Degrees to Radians/1
  Add/1 -> [alpha_fault_free_rad]
  Constant1/1 -> [bias_fault_active]
  Constant2/1 -> [drift_fault_active]
  [bias_fault_active] -> Enabled Subsystem/Enable
  [alpha_fault_free_rad] -> Enabled Subsystem/1(alpha_fault_free)
  [drift_fault_active] -> Enabled Subsystem1/Enable
  [alpha_fault_free_rad] -> Enabled Subsystem1/1(alpha_fault_free)
  Enabled Subsystem/1(alpha_biased_rad) -> [alpha_biased_rad]
  Enabled Subsystem1/1(alpha_drifted_rad) -> [alpha_drifted_rad]
  [alpha_biased_rad] -> MATLAB Function/3(alpha_biased_rad)
  [bias_fault_active] -> MATLAB Function/2(bias_fault_active)
  [drift_fault_active] -> MATLAB Function/4(drift_fault_active)
  [alpha_drifted_rad] -> MATLAB Function/5(alpha_drifted_rad)
  [alpha_fault_free_rad] -> MATLAB Function/1(alpha_fault_free_rad)
  MATLAB Function/1(y) -> [alpha_measurement_rad]
  [alpha_measurement_rad] -> alpha_measurement_rad/1
  Degrees to Radians/1 -> Add/2
  Constant3/1 -> [stuck_fault_active]

== system aerosonde_dynamics_with_autopilot/Distance Travelled Calculator ==
  X Coordinate : Inport
  Y Coordinate : Inport  Port=2
  Z coordinate : Inport  Port=3
  Delay X : Delay  DelayLength=1  InitialCondition=flightconfig.position_0(1)
  Delay Y : Delay  DelayLength=1  InitialCondition=flightconfig.position_0(2)
  Delay Z : Delay  DelayLength=1  InitialCondition=flightconfig.position_0(3)
  Distance last step : Delay  DelayLength=1  InitialCondition=flightconfig.distance_travelled
  Math Function : Math  Operator=magnitude^2  SignedPower=on  SaturateOnIntegerOverflow=on
  Math Function1 : Math  Operator=magnitude^2  SignedPower=on  SaturateOnIntegerOverflow=on
  Math Function2 : Math  Operator=magnitude^2  SignedPower=on  SaturateOnIntegerOverflow=on
  Sqrt : Sqrt  SaturateOnIntegerOverflow=on
  Sum : Sum  Inputs=|+-
  Sum1 : Sum  Inputs=|+++
  Sum2 : Sum  Inputs=|+-
  Sum3 : Sum  Inputs=|+-
  Sum4 : Sum  Inputs=|++
  Distance_travelled : Outport
  wires:
  Delay X/1 -> Sum/2
  Sum/1 -> Math Function/1
  Math Function/1 -> Sum1/1
  Delay Y/1 -> Sum2/2
  Sum2/1 -> Math Function1/1
  Math Function1/1 -> Sum1/2
  Delay Z/1 -> Sum3/2
  Sum3/1 -> Math Function2/1
  Math Function2/1 -> Sum1/3
  Sum1/1 -> Sqrt/1
  Sqrt/1 -> Sum4/1
  Distance last step/1 -> Sum4/2
  Sum4/1 -> Distance_travelled/1, Distance last step/1  "Fuel_mass_out"
  Z coordinate/1 -> Sum3/1, Delay Z/1
  X Coordinate/1 -> Sum/1, Delay X/1
  Y Coordinate/1 -> Sum2/1, Delay Y/1

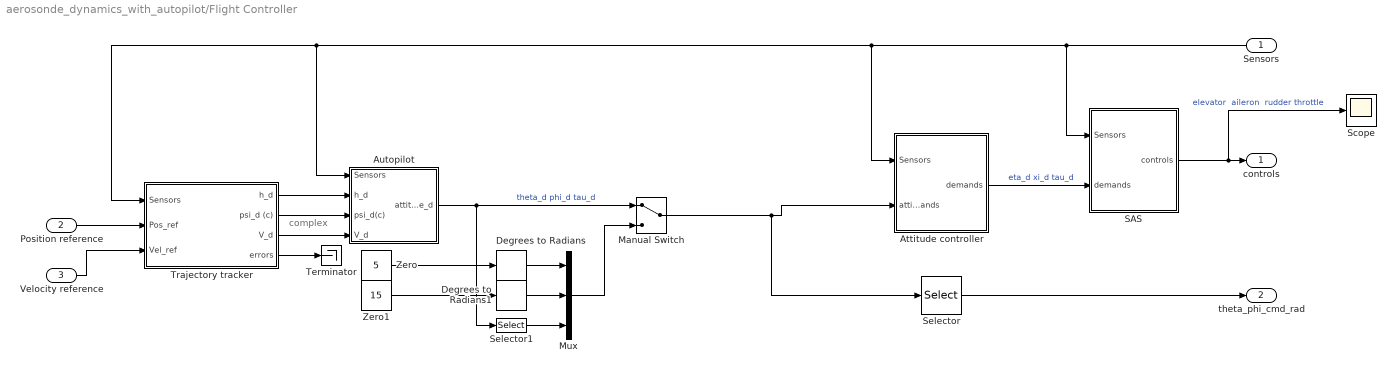
== system aerosonde_dynamics_with_autopilot/Flight Controller ==
  note: complex
  Sensors : Inport
  Position reference : Inport  Port=2
  Velocity reference : Inport  Port=3
  Attitude controller : Subsystem
  Autopilot : Subsystem
  Degrees to Radians : simulink_extras/Transformations/Degrees to Radians
  Degrees to Radians1 : simulink_extras/Transformations/Degrees to Radians
  Manual Switch : ManualSwitch
  Mux : Mux  Inputs=3
  SAS : Subsystem
  Scope : Scope
  Selector : Selector  InputPortWidth=3  IndexOptions=Index vector (dialog)  Indices=[1 2]  OutputSizes=1
  Selector1 : Selector  InputPortWidth=3  IndexOptions=Index vector (dialog)  Indices=[3]  OutputSizes=1
  Terminator : Terminator
  Trajectory tracker : Subsystem
  Zero : Constant  Value=5  OutDataTypeStr=Inherit: Inherit via back propagation
  Zero1 : Constant  Value=15  OutDataTypeStr=Inherit: Inherit via back propagation
  controls : Outport
  theta_phi_cmd_rad : Outport  Port=2
  wires:
  Sensors/1 -> SAS/1(Sensors), Attitude controller/1(Sensors), Autopilot/1(Sensors), Trajectory tracker/1(Sensors)
  Attitude controller/1(demands) -> SAS/2(demands)  "eta_d xi_d tau_d"
  SAS/1(controls) -> Scope/1, controls/1  "elevator  aileron  rudder throttle"
  Trajectory tracker/2(psi_d (c)) -> Autopilot/3(psi_d(c))
  Position reference/1 -> Trajectory tracker/2(Pos_ref)
  Velocity reference/1 -> Trajectory tracker/3(Vel_ref)
  Trajectory tracker/4(errors) -> Terminator/1
  Trajectory tracker/1(h_d) -> Autopilot/2(h_d)
  Trajectory tracker/3(V_d) -> Autopilot/4(V_d)
  Selector/1 -> theta_phi_cmd_rad/1
  Selector1/1 -> Mux/3
  Autopilot/1(attitude_d) -> Manual Switch/1, Selector1/1  "theta_d phi_d tau_d"
  Degrees to Radians/1 -> Mux/1
  Zero/1 -> Degrees to Radians/1
  Degrees to Radians1/1 -> Mux/2
  Zero1/1 -> Degrees to Radians1/1
  Mux/1 -> Manual Switch/2
  Manual Switch/1 -> Selector/1, Attitude controller/2(attitude demands)

== system aerosonde_dynamics_with_autopilot/Stop Conditions ==
  Altitude : Inport
  Fuel_Remaining : Inport  Port=2
  Distance_ Travelled : Inport  Port=3
  Clock1 : Clock
  Compare To Constant1 : simulink/Logic and Bit Operations/Compare To Constant  relop=>  const=flightconfig.segment_length  OutDataTypeStr=boolean
  Compare To Constant2 : simulink/Logic and Bit Operations/Compare To Constant  relop=>  const=flightconfig.mission_segment_distance  OutDataTypeStr=boolean
  Compare To Zero1 : simulink/Logic and Bit Operations/Compare To Zero  relop=<  OutDataTypeStr=boolean
  Compare To Zero2 : simulink/Logic and Bit Operations/Compare To Zero  relop=<  OutDataTypeStr=boolean
  Stop Simulation{,1..3} (4 alike) : Stop
  Transport Delay1 : TransportDelay  DelayTime=100  InitialOutput=-flightconfig.position_0(3)  BufferSize=5048  FixedBuffer=on  TransDelayFeedthrough=on
  Transport Delay2 : TransportDelay  DelayTime=1000  InitialOutput=flightconfig.fuel_0  BufferSize=5048  FixedBuffer=on  TransDelayFeedthrough=on
  Transport Delay3 : TransportDelay  DelayTime=100  InitialOutput=flightconfig.distance_travelled  BufferSize=5048  FixedBuffer=on  TransDelayFeedthrough=on
  wires:
  Distance_ Travelled/1 -> Transport Delay3/1
  Altitude/1 -> Transport Delay1/1
  Fuel_Remaining/1 -> Transport Delay2/1
  Transport Delay1/1 -> Compare To Zero1/1
  Compare To Zero1/1 -> Stop Simulation1/1  "Altitude_zero_flag"
  Transport Delay2/1 -> Compare To Zero2/1
  Compare To Zero2/1 -> Stop Simulation/1  "fuel_zero_flag"
  Clock1/1 -> Compare To Constant1/1
  Compare To Constant1/1 -> Stop Simulation2/1
  Transport Delay3/1 -> Compare To Constant2/1
  Compare To Constant2/1 -> Stop Simulation3/1  "mission_distance_completed_flag"

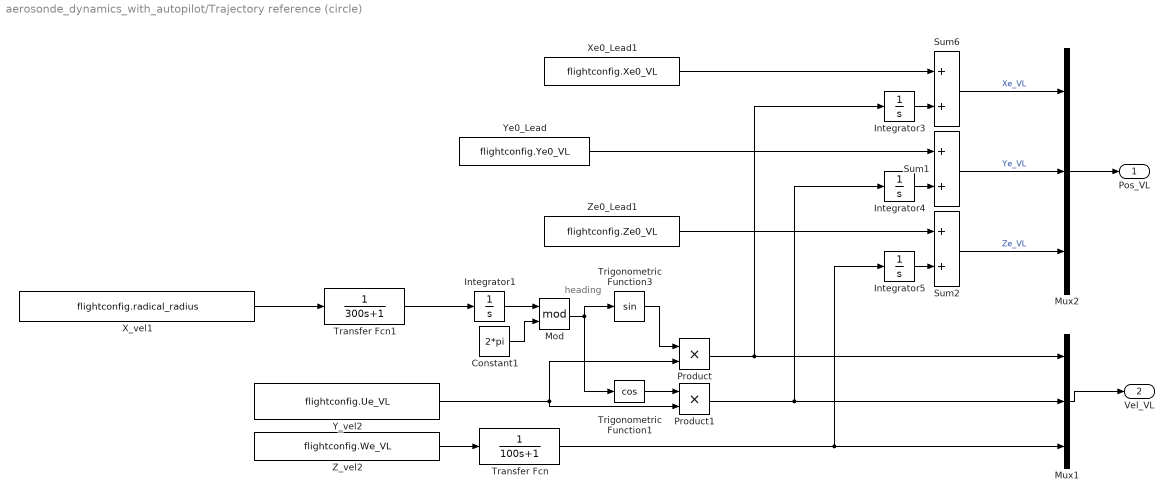
== system aerosonde_dynamics_with_autopilot/Trajectory reference (circle) ==
  note: heading
  Constant1 : Constant  Value=2*pi
  Integrator{1,3..5} (4 alike) : Integrator
  Mod : Math  Operator=mod  SaturateOnIntegerOverflow=on
  Mux1 : Mux  Inputs=3
  Mux2 : Mux  Inputs=3
  Product : Product  RndMeth=Zero
  Product1 : Product  RndMeth=Zero
  Sum1 : Sum
  Sum2 : Sum
  Sum6 : Sum
  Transfer Fcn : TransferFcn  Denominator=[100 1]
  Transfer Fcn1 : TransferFcn  Denominator=[300 1]
  Trigonometric Function1 : Trigonometry  Operator=cos
  Trigonometric Function3 : Trigonometry
  X_vel1 : Constant  Value=flightconfig.radical_radius
  Xe0_Lead1 : Constant  Value=flightconfig.Xe0_VL  VectorParams1D=off
  Y_vel2 : Constant  Value=flightconfig.Ue_VL
  Ye0_Lead : Constant  Value=flightconfig.Ye0_VL
  Z_vel2 : Constant  Value=flightconfig.We_VL
  Ze0_Lead1 : Constant  Value=flightconfig.Ze0_VL
  Pos_VL : Outport
  Vel_VL : Outport  Port=2
  wires:
  Trigonometric Function1/1 -> Product1/1
  Mod/1 -> Trigonometric Function1/1, Trigonometric Function3/1
  Trigonometric Function3/1 -> Product/1
  Product1/1 -> Integrator4/1, Mux1/2
  Product/1 -> Integrator3/1, Mux1/1
  Transfer Fcn/1 -> Integrator5/1, Mux1/3
  Mux1/1 -> Vel_VL/1
  Y_vel2/1 -> Product1/2, Product/2
  Ye0_Lead/1 -> Sum1/1
  Xe0_Lead1/1 -> Sum6/1
  Ze0_Lead1/1 -> Sum2/1
  Integrator3/1 -> Sum6/2
  Integrator4/1 -> Sum1/2
  Integrator5/1 -> Sum2/2
  Sum2/1 -> Mux2/3  "Ze_VL"
  Sum1/1 -> Mux2/2  "Ye_VL"
  Sum6/1 -> Mux2/1  "Xe_VL"
  Mux2/1 -> Pos_VL/1
  Integrator1/1 -> Mod/1
  Constant1/1 -> Mod/2
  Z_vel2/1 -> Transfer Fcn/1
  X_vel1/1 -> Transfer Fcn1/1
  Transfer Fcn1/1 -> Integrator1/1

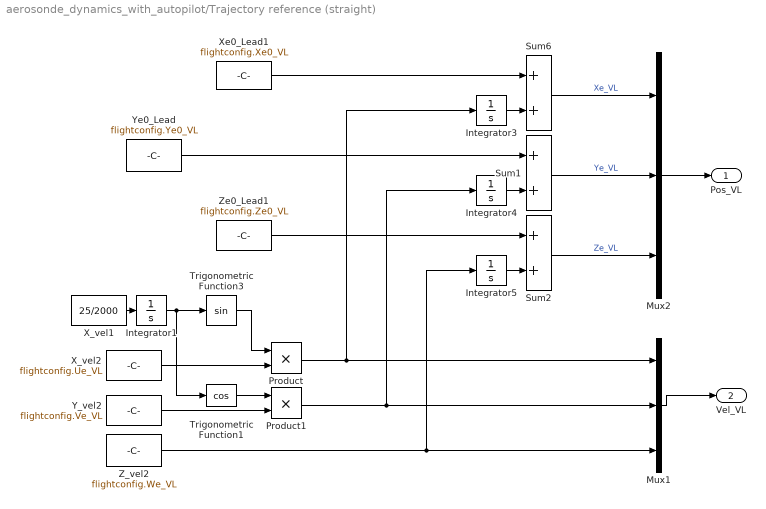
== system aerosonde_dynamics_with_autopilot/Trajectory reference (straight) ==
  Integrator{1,3..5} (4 alike) : Integrator
  Mux1 : Mux  Inputs=3
  Mux2 : Mux  Inputs=3
  Product : Product  RndMeth=Zero
  Product1 : Product  RndMeth=Zero
  Sum1 : Sum
  Sum2 : Sum
  Sum6 : Sum
  Trigonometric Function1 : Trigonometry  Operator=cos
  Trigonometric Function3 : Trigonometry
  X_vel1 : Constant  Value=25/2000
  X_vel2 : Constant  Value=flightconfig.Ue_VL
  Xe0_Lead1 : Constant  Value=flightconfig.Xe0_VL
  Y_vel2 : Constant  Value=flightconfig.Ve_VL
  Ye0_Lead : Constant  Value=flightconfig.Ye0_VL
  Z_vel2 : Constant  Value=flightconfig.We_VL
  Ze0_Lead1 : Constant  Value=flightconfig.Ze0_VL
  Pos_VL : Outport
  Vel_VL : Outport  Port=2
  wires:
  Sum6/1 -> Mux2/1  "Xe_VL"
  Sum1/1 -> Mux2/2  "Ye_VL"
  Sum2/1 -> Mux2/3  "Ze_VL"
  Mux2/1 -> Pos_VL/1
  Integrator5/1 -> Sum2/2
  Integrator4/1 -> Sum1/2
  Integrator3/1 -> Sum6/2
  Ze0_Lead1/1 -> Sum2/1
  Xe0_Lead1/1 -> Sum6/1
  Ye0_Lead/1 -> Sum1/1
  X_vel2/1 -> Product/2
  Y_vel2/1 -> Product1/2
  Mux1/1 -> Vel_VL/1
  Z_vel2/1 -> Mux1/3, Integrator5/1
  Product/1 -> Mux1/1, Integrator3/1
  Product1/1 -> Mux1/2, Integrator4/1
  Trigonometric Function3/1 -> Product/1
  X_vel1/1 -> Integrator1/1
  Integrator1/1 -> Trigonometric Function3/1, Trigonometric Function1/1
  Trigonometric Function1/1 -> Product1/1

== system aerosonde_dynamics_with_autopilot/Wind Model ==
  note: Wind Models
  altitude h (m) : Inport
  DCM : Inport  Port=2
  V_E (m/s) : Inport  Port=3
  Dot Product : DotProduct  SaturateOnIntegerOverflow=on  OutDataTypeStr=Inherit: Inherit via internal rule
  Dryden Wind Turbulence Model (Continuous (+q +r)) : aerolibwind2/Dryden Wind Turbulence Model  (Continuous (+q -r))  units=Metric (MKS)  spec=MIL-F-8785C  model=Continuous Von Karman (+q -r)  W20=0  Wdeg=90  TurbProb=2x10^-1  L_high=533.4  Wingspan=aerosonde.b  ts=0.02  Seed=[23341 23342 23343 23344]  T_on=on
  Horizontal Wind Model : aerolibwind2/Horizontal Wind Model  units=Metric (MKS)  Vw_source=Internal  Vwind=0  W_source=Internal  Wdeg=-60
      settings: SourceProductBaseCode=AE
  Sum : Sum  Inputs=+++  InputSameDT=on  SaturateOnIntegerOverflow=on  OutDataTypeStr=Inherit: Same as first input
  V : Math  Operator=sqrt  SignedPower=on  SaturateOnIntegerOverflow=on
  Wind Shear Model : aerolibwind2/Wind Shear Model  units=Metric (MKS)  phase=Category C - Terminal Flight Phase  W_20=0  Wdeg=0
  ground speed1 : Scope
  V_wind : Outport
  omega_wind : Outport  Port=2
  wires:
  Wind Shear Model/1 -> Sum/1
  Horizontal Wind Model/1 -> Sum/2
  altitude h (m)/1 -> Wind Shear Model/1, Dryden Wind Turbulence Model (Continuous (+q +r))/1
  DCM/1 -> Wind Shear Model/2, Dryden Wind Turbulence Model (Continuous (+q +r))/3, Horizontal Wind Model/1
  Sum/1 -> V_wind/1
  Dryden Wind Turbulence Model (Continuous (+q +r))/2 -> omega_wind/1
  Dot Product/1 -> V/1
  V_E (m/s)/1 -> Dot Product/1, Dot Product/2
  Dryden Wind Turbulence Model (Continuous (+q +r))/1 -> Sum/3
  V/1 -> Dryden Wind Turbulence Model (Continuous (+q +r))/2, ground speed1/1

== system aerosonde_dynamics_with_autopilot/ UAV Dynamics/Aerodynamics ==
  note: Aerodynamic Model
  note: Aerodynamic Coefficients
  note: Aerodynamic Parameters
  note: Outputs
  note: Inputs
  VelB : Inport  PortDimensions=[3 1]
  WindB : Inport  Port=2  PortDimensions=[3 1]
  VelBdot : Inport  Port=3
  Rates : Inport  Port=4  PortDimensions=[3 1]
  WindRates : Inport  Port=5  PortDimensions=[3 1]
  AeroCon : Inport  Port=6  PortDimensions=[4 1]
  rho : Inport  Port=7  PortDimensions=1
  "a " : Inport  Port=8  PortDimensions=1
  Force Coefficients : Subsystem
  Moment Coefficients : Subsystem
  Mux : Mux  Inputs=2
  Sum : Sum  Inputs=|+-  InputSameDT=on  SaturateOnIntegerOverflow=on  OutDataTypeStr=Inherit: Same as first input
  Wind-axes Velocities : Subsystem
  AeroCoeff_ba : Outport
  VelW : Outport  Port=2
  Mach : Outport  Port=3
  qbar (pdyn) : Outport  Port=4
  wires:
  VelBdot/1 -> Wind-axes Velocities/5(VelBdot)
  Wind-axes Velocities/4(alphadot) -> Force Coefficients/3(AlphaDot), Moment Coefficients/3(AlphaDot)
  WindB/1 -> Wind-axes Velocities/2(WindB)
  Mux/1 -> AeroCoeff_ba/1
  Moment Coefficients/1("[-Cl, Cm, -Cn]") -> Mux/2
  Force Coefficients/1("[-CD, CY, -CL]") -> Mux/1
  rho/1 -> Wind-axes Velocities/4(rho)
  VelB/1 -> Wind-axes Velocities/1(VelB)
  "a "/1 -> Wind-axes Velocities/3(a)  "speed of sound"
  Wind-axes Velocities/1(VBetaAlpha) -> Moment Coefficients/1(VBetaAlpha), VelW/1, Force Coefficients/1(VBetaAlpha)
  AeroCon/1 -> Moment Coefficients/2(Control), Force Coefficients/2(Control)
  Wind-axes Velocities/2(Mach) -> Mach/1, Moment Coefficients/5(Mach), Force Coefficients/5(Mach)
  Wind-axes Velocities/3(qbar (pdyn)) -> qbar (pdyn)/1
  Rates/1 -> Sum/1
  WindRates/1 -> Sum/2
  Sum/1 -> Moment Coefficients/4(AngularRates), Force Coefficients/4(AngularRates)  "pqr"

== system aerosonde_dynamics_with_autopilot/ UAV Dynamics/Aircraft Mass & Inertia ==
  note: Compute current aircraft mass
  FuelFlow : Inport  PortDimensions=1
  RST : Inport  Port=2  PortDimensions=1
  ChSign : Gain  Gain=-1  SaturateOnIntegerOverflow=on  OutDataTypeStr=Inherit: Same as input  ParamDataTypeStr=Inherit: Same as input
  Estimate Center of Gravity : aerolibbdyn/Estimate Center of Gravity  fmass=aerosonde.mgross  emass=aerosonde.mempty  fcg=aerosonde.CGgross  ecg=aerosonde.CGempty
      settings: SourceProductBaseCode=AE
  Estimate Inertia Tensor : shareddyn/Estimate Inertia Tensor  fmass=aerosonde.mgross  emass=aerosonde.mempty  fI=aerosonde.J_gross  eI=aerosonde.J_empty  aMode=aMode
      settings: SourceProductBaseCode=AE,PW,DR,MT,UV,VE
  Fuel Integrator : Integrator  ExternalReset=rising  InitialCondition=flightconfig.fuel_0  LimitOutput=on  UpperSaturationLimit=aerosonde.mgross-aerosonde.mempty  LowerSaturationLimit=0
  Mass empty : Constant  Value=aerosonde.mempty
  Relational Operator : RelationalOperator  Operator===  RndMeth=Nearest  InputSameDT=on
  Sum : Sum  Inputs=|++  InputSameDT=on  SaturateOnIntegerOverflow=on  OutDataTypeStr=Inherit: Same as first input
  Mass : Outport
  mdot : Outport  Port=2
  Inertia : Outport  Port=3
  Inertiadot : Outport  Port=4
  CGpos : Outport  Port=5
  CGposdot : Outport  Port=6
  Fuel : Outport  Port=7
  OutofFuel : Outport  Port=8
  wires:
  Estimate Center of Gravity/2 -> CGposdot/1
  Estimate Center of Gravity/1 -> CGpos/1
  Estimate Inertia Tensor/2 -> Inertiadot/1
  Estimate Inertia Tensor/1 -> Inertia/1
  Sum/1 -> Relational Operator/1, Estimate Center of Gravity/1, Estimate Inertia Tensor/1, Mass/1
  Mass empty/1 -> Sum/2, Relational Operator/2
  Fuel Integrator/1 -> Sum/1, Fuel/1
  RST/1 -> Fuel Integrator/2
  ChSign/1 -> Estimate Center of Gravity/2, Estimate Inertia Tensor/2, mdot/1, Fuel Integrator/1
  FuelFlow/1 -> ChSign/1
  Relational Operator/1 -> OutofFuel/1

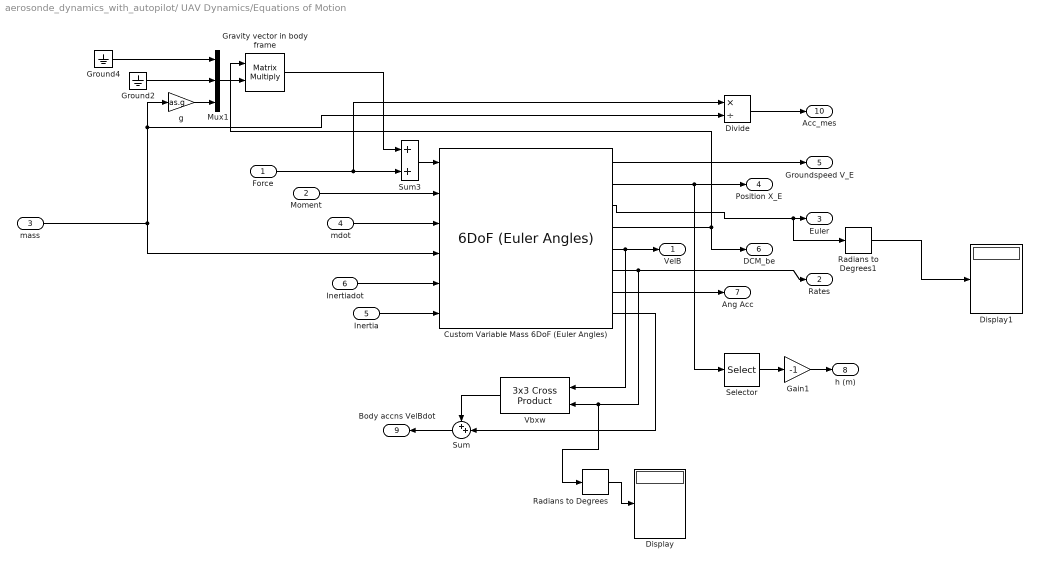
== system aerosonde_dynamics_with_autopilot/ UAV Dynamics/Equations of Motion ==
  Force : Inport  PortDimensions=3
  Moment : Inport  Port=2  PortDimensions=3
  mass : Inport  Port=3  PortDimensions=1
  mdot : Inport  Port=4  PortDimensions=1
  Inertia : Inport  Port=5  PortDimensions=[3,3]
  Inertiadot : Inport  Port=6  PortDimensions=[3,3]
  Custom Variable Mass 6DoF (Euler Angles) : aerolibobsolete/6DoF (Euler Angles)  units=Metric (MKS)  mtype=Custom Variable  rep=Euler Angles  xme_0=flightconfig.position_0  Vm_0=flightconfig.velocity_0  eul_0=flightconfig.euler_0  pm_0=flightconfig.rates_0  mass_0=1.0  mass_e=0  mass_f=0  inertia=eye(3)  inertia_e=eye(3)  inertia_f=eye(3)  k_quat=1.0
      settings: SourceProductBaseCode=AE
  Display : Display
  Display1 : Display
  Divide : Product  Inputs=*/
  Gain1 : Gain  Gain=-1
  "Gravity vector in body frame " : Product  Multiplication=Matrix(*)  InputSameDT=on  SaturateOnIntegerOverflow=on  OutDataTypeStr=Inherit: Same as first input
  Ground2 : Ground
  Ground4 : Ground
  Mux1 : Mux  Inputs=3
  Radians to Degrees : simulink_extras/Transformations/Radians to Degrees
  Radians to Degrees1 : simulink_extras/Transformations/Radians to Degrees
  Selector : Selector  InputPortWidth=3  IndexOptions=Index vector (dialog)  Indices=3  OutputSizes=1
  Sum : Sum  Inputs=++|  SaturateOnIntegerOverflow=on
  Sum3 : Sum  InputSameDT=on  SaturateOnIntegerOverflow=on  OutDataTypeStr=Inherit: Same as first input
  Vbxw : sharedutil/3x3 Cross Product  aMode=aMode
      settings: SourceProductBaseCode=AE,PW,DR,MT,UV,VE
  g : Gain  Gain=as.g
  VelB : Outport
  Rates : Outport  Port=2
  Euler : Outport  Port=3
  Position X_E : Outport  Port=4
  Groundspeed V_E : Outport  Port=5
  DCM_be : Outport  Port=6
  Ang Acc : Outport  Port=7
  h (m) : Outport  Port=8
  Body accns VelBdot : Outport  Port=9
  Acc_mes : Outport  Port=10
  wires:
  Vbxw/1 -> Sum/1
  Sum/1 -> Body accns VelBdot/1
  Custom Variable Mass 6DoF (Euler Angles)/8 -> Sum/2
  Custom Variable Mass 6DoF (Euler Angles)/7 -> Ang Acc/1
  Custom Variable Mass 6DoF (Euler Angles)/6 -> Radians to Degrees/1, Vbxw/2, Rates/1
  Inertia/1 -> Custom Variable Mass 6DoF (Euler Angles)/6
  mdot/1 -> Custom Variable Mass 6DoF (Euler Angles)/3
  Inertiadot/1 -> Custom Variable Mass 6DoF (Euler Angles)/5
  Gain1/1 -> h (m)/1
  Selector/1 -> Gain1/1
  Sum3/1 -> Custom Variable Mass 6DoF (Euler Angles)/1
  g/1 -> Mux1/3
  "Gravity vector in body frame "/1 -> Sum3/1
  Custom Variable Mass 6DoF (Euler Angles)/3 -> Radians to Degrees1/1, Euler/1
  Custom Variable Mass 6DoF (Euler Angles)/2 -> Selector/1, Position X_E/1
  Custom Variable Mass 6DoF (Euler Angles)/1 -> Groundspeed V_E/1
  Custom Variable Mass 6DoF (Euler Angles)/5 -> Vbxw/1, VelB/1
  Ground4/1 -> Mux1/1
  Ground2/1 -> Mux1/2
  Custom Variable Mass 6DoF (Euler Angles)/4 -> DCM_be/1, "Gravity vector in body frame "/1
  Mux1/1 -> "Gravity vector in body frame "/2
  Force/1 -> Divide/1, Sum3/2
  Moment/1 -> Custom Variable Mass 6DoF (Euler Angles)/2
  Radians to Degrees/1 -> Display/1
  Radians to Degrees1/1 -> Display1/1
  mass/1 -> Custom Variable Mass 6DoF (Euler Angles)/4, Divide/2, g/1
  Divide/1 -> Acc_mes/1

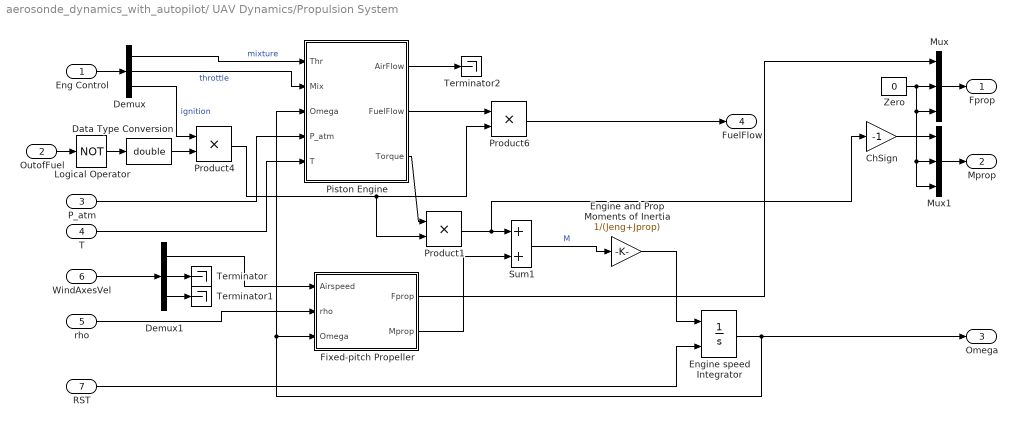
== system aerosonde_dynamics_with_autopilot/ UAV Dynamics/Propulsion System ==
  Eng Control : Inport  PortDimensions=[3 1]
  OutofFuel : Inport  Port=2  PortDimensions=1
  P_atm : Inport  Port=3  OutDataTypeStr=double  PortDimensions=1
  T : Inport  Port=4  OutDataTypeStr=double  PortDimensions=1
  rho : Inport  Port=5  OutDataTypeStr=double  PortDimensions=1
  WindAxesVel : Inport  Port=6  PortDimensions=[3 1]
  RST : Inport  Port=7  OutDataTypeStr=double  PortDimensions=1
  ChSign : Gain  Gain=-1  SaturateOnIntegerOverflow=on  OutDataTypeStr=Inherit: Same as input  ParamDataTypeStr=Inherit: Same as input
  Data Type Conversion : DataTypeConversion  OutDataTypeStr=double  SaturateOnIntegerOverflow=on  RndMeth=Zero
  Demux : Demux  Outputs=3
      settings: DisplayOption=none
  Demux1 : Demux  Outputs=3
      settings: DisplayOption=none
  Engine and Prop Moments of Inertia : Gain  Gain=1/(Jeng+Jprop)  SaturateOnIntegerOverflow=on  OutDataTypeStr=Inherit: Same as input  ParamDataTypeStr=Inherit: Same as input
  Engine speed Integrator : Integrator  ExternalReset=rising  InitialCondition=OmegaIni  LimitOutput=on  LowerSaturationLimit=0
  Fixed-pitch Propeller : Subsystem
  Logical Operator : Logic  Operator=NOT
  Mux : Mux  Inputs=3
  Mux1 : Mux  Inputs=3
  Piston Engine : Subsystem  mask(Piston Engine){RPM=RPM, MAP=MAP, fflow=FuelFlow, Power=Power, TSL=TSL}
      mask prompts: RPM "RPM vector:"; MAP "MAP vector:"; fflow "Fuel flow 2-D look-up table:"; Power "Power 2-D look-up table:"; TSL "Sea-level temperature:"
      mask help: The piston engine model computes the engine parameters at current throttle setting, engine rpm, and altitude.
      mask Help:
      | The block provides a piston engine model based on look-up tables for manifold pressure, engine speed (rpm), fuel flow and power.
      | <P><B>Inputs:</B>
      | <LI>Thr = the throttle command (as a fraction of atmospheric pressure)</LI>
      | <LI>Mix = the air to fuel mixture ratio</LI>
      | <LI>Omega = the engine shaft rotation speed</LI>
      | <LI>p = the atmospheric pressure, in Pa</LI>
      | <LI>T = the atmospheric temperature, in K</LI>
      | </P>
      | <P><B>Output:</B>
      | <LI>MAP = the manifold air pressure, in kPa</LI>
      | <LI>AirFlow = the mass air flow, in kg/s</LI>
      | <LI>FuelFlow = the mass fuel flow, in kg/s</LI>
      | <LI>BSFC = the brake-specific fuel consumption, in g/(W*hr)</LI>
      | <LI>Power = the engine power, in W</LI>
      | <LI>Torque = the engine shaft torque, in N*m</LI>
      | </P>
      | <P><B>Parameters:</B>
      | <LI>RPM vector = the engine speed interpolation vector, in rpm</LI>
      | <LI>MAP vector = the manifold air pressure interpolation vector, in kPa</LI>
      | <LI>Fuel flow = the 2-D look-up table for fuel flow, as function of MAP and RPM, in g/hr</LI>
      | <LI>Power = the 2-D look-up table for power, as function of MAP and RPM, in W</LI>
      | <LI>Sea-level temperature = the ambient temperature for which the above engine look-up tables are given</LI>
      | </P>
  Product1 : Product  InputSameDT=on  SaturateOnIntegerOverflow=on  OutDataTypeStr=Inherit: Same as first input
  Product4 : Product  InputSameDT=on  SaturateOnIntegerOverflow=on  OutDataTypeStr=Inherit: Same as first input
  Product6 : Product  InputSameDT=on  SaturateOnIntegerOverflow=on  OutDataTypeStr=Inherit: Same as first input
  Sum1 : Sum  InputSameDT=on  SaturateOnIntegerOverflow=on  OutDataTypeStr=Inherit: Same as first input
  Terminator : Terminator
  Terminator1 : Terminator
  Terminator2 : Terminator
  Zero : Constant  Value=0
  Fprop : Outport
  Mprop : Outport  Port=2
  Omega : Outport  Port=3
  FuelFlow : Outport  Port=4
  wires:
  Piston Engine/1(AirFlow) -> Terminator2/1
  Product6/1 -> FuelFlow/1
  Piston Engine/2(FuelFlow) -> Product6/1
  Engine and Prop Moments of Inertia/1 -> Engine speed Integrator/1
  T/1 -> Piston Engine/5(T)
  P_atm/1 -> Piston Engine/4(P_atm)
  Demux/2 -> Piston Engine/2(Mix)  "throttle"
  Demux/3 -> Product4/1  "ignition"
  Logical Operator/1 -> Data Type Conversion/1
  Mux1/1 -> Mprop/1
  Mux/1 -> Fprop/1
  ChSign/1 -> Mux1/1
  Zero/1 -> Mux1/2, Mux1/3, Mux/3, Mux/2
  Piston Engine/3(Torque) -> Product1/1
  Engine speed Integrator/1 -> Omega/1, Piston Engine/3(Omega), Fixed-pitch Propeller/3(Omega)
  RST/1 -> Engine speed Integrator/2
  Sum1/1 -> Engine and Prop Moments of Inertia/1  "M"
  Product1/1 -> ChSign/1, Sum1/1
  Product4/1 -> Product1/2, Product6/2
  OutofFuel/1 -> Logical Operator/1
  rho/1 -> Fixed-pitch Propeller/2(rho)
  Demux1/1 -> Fixed-pitch Propeller/1(Airspeed)
  Demux1/3 -> Terminator1/1
  Demux1/2 -> Terminator/1
  WindAxesVel/1 -> Demux1/1
  Eng Control/1 -> Demux/1
  Data Type Conversion/1 -> Product4/2
  Fixed-pitch Propeller/1(Fprop) -> Mux/1
  Fixed-pitch Propeller/2(Mprop) -> Sum1/2
  Demux/1 -> Piston Engine/1(Thr)  "mixture"
